simulink model "hexGroundContactTestHarness"  (R2024a)
settings: configuration reference "standardSILConfiguraitonParams" (kept outside this file)
undefined symbols (not defined in the file): vehicleParams
settings Model: Creator=jerem  LastModifiedBy=jerem
settings ConfigSetRef: SourceName=standardSILConfiguraitonParams  SourceLocation=Base Workspace

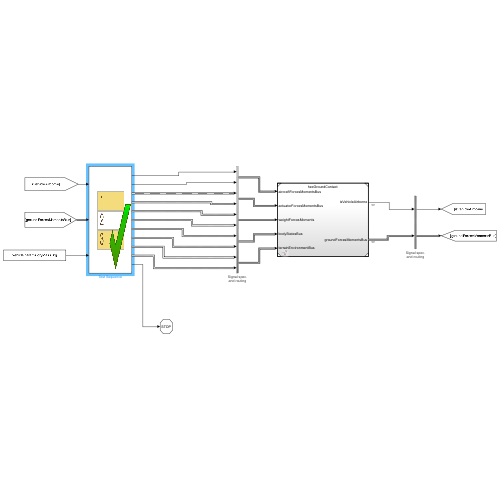
[thumbnail: Simulink's stored preview of the top-level diagram]
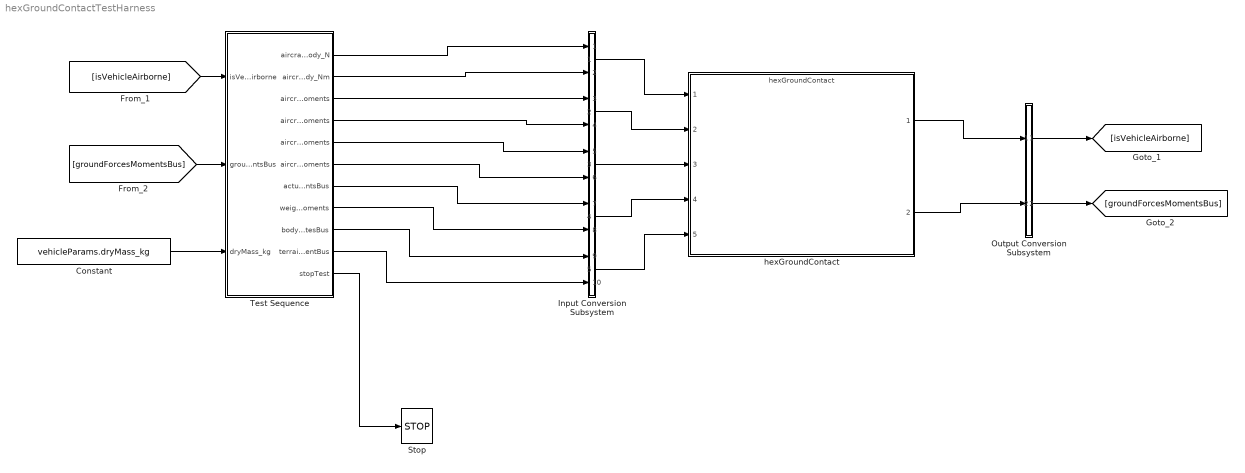
== system hexGroundContactTestHarness ==
  Constant : Constant  Value=vehicleParams.dryMass_kg
  Input Conversion Subsystem : Subsystem  Tag=__SLT_ICS__  Description=|
      | Signal spec.
      | and routing
      settings: AttributesFormatString=%<Description>
  Output Conversion Subsystem : Subsystem  Tag=__SLT_OCS__  Description=|
      | Signal spec.
      | and routing
      mask init:
      | ICDictionary = get_param(bdroot, 'DataDictionary');
      | if isempty(ICDictionary)
      |    ICScope = Simulink.data.BaseWorkspace;
      | else
      |    ICScope = Simulink.data.DataDictionary(ICDictionary);
      | end
      | 
      | IC2 = Simulink.Bus.createMATLABStruct('ComponentForcesMomentsBus', [], [1 1], ICScope);
      settings: AttributesFormatString=%<Description>
  Stop : Stop
  Test Sequence : Test Sequence  TreatAsAtomicUnit=on
  hexGroundContact : ModelReference  ModelNameDialog=hexGroundContact  SimulationMode=Normal  ModelReferenceVersion=1.58
  wires:
  Test Sequence/1(aircraftForcesMomentsBus_forcesInBody_N) -> Input Conversion Subsystem/1(Inport_1)
  Test Sequence/2(aircraftForcesMomentsBus_momentsInBody_Nm) -> Input Conversion Subsystem/2(Inport_2)
  Test Sequence/3(aircraftForcesMomentsBus_aeroForcesMoments) -> Input Conversion Subsystem/3(Inport_3)
  Test Sequence/4(aircraftForcesMomentsBus_engineForcesMoments) -> Input Conversion Subsystem/4(Inport_4)
  Test Sequence/5(aircraftForcesMomentsBus_groundForcesMoments) -> Input Conversion Subsystem/5(Inport_5)
  Test Sequence/6(aircraftForcesMomentsBus_weightForcesMoments) -> Input Conversion Subsystem/6(Inport_6)
  Test Sequence/7(actuatorForcesMomentsBus) -> Input Conversion Subsystem/7(Inport_7)
  Test Sequence/8(weightForcesMoments) -> Input Conversion Subsystem/8(Inport_8)
  Test Sequence/9(bodyStatesBus) -> Input Conversion Subsystem/9(Inport_9)
  Test Sequence/10(terrainEnvironmentBus) -> Input Conversion Subsystem/10(Inport_10)
  [isVehicleAirborne] -> Test Sequence/1(isVehicleAirborne)
  [groundForcesMomentsBus] -> Test Sequence/2(groundForcesMomentsBus)
  Output Conversion Subsystem/1(Outport_1) -> [isVehicleAirborne]
  Output Conversion Subsystem/2(Outport_2) -> [groundForcesMomentsBus]
  Input Conversion Subsystem/1(Outport_1) -> hexGroundContact/1
  Input Conversion Subsystem/2(Outport_2) -> hexGroundContact/2
  Input Conversion Subsystem/3(Outport_3) -> hexGroundContact/3
  Input Conversion Subsystem/4(Outport_4) -> hexGroundContact/4
  Input Conversion Subsystem/5(Outport_5) -> hexGroundContact/5
  hexGroundContact/1 -> Output Conversion Subsystem/1(Inport_1)
  hexGroundContact/2 -> Output Conversion Subsystem/2(Inport_2)
  Test Sequence/11(stopTest) -> Stop/1
  Constant/1 -> Test Sequence/3(dryMass_kg)

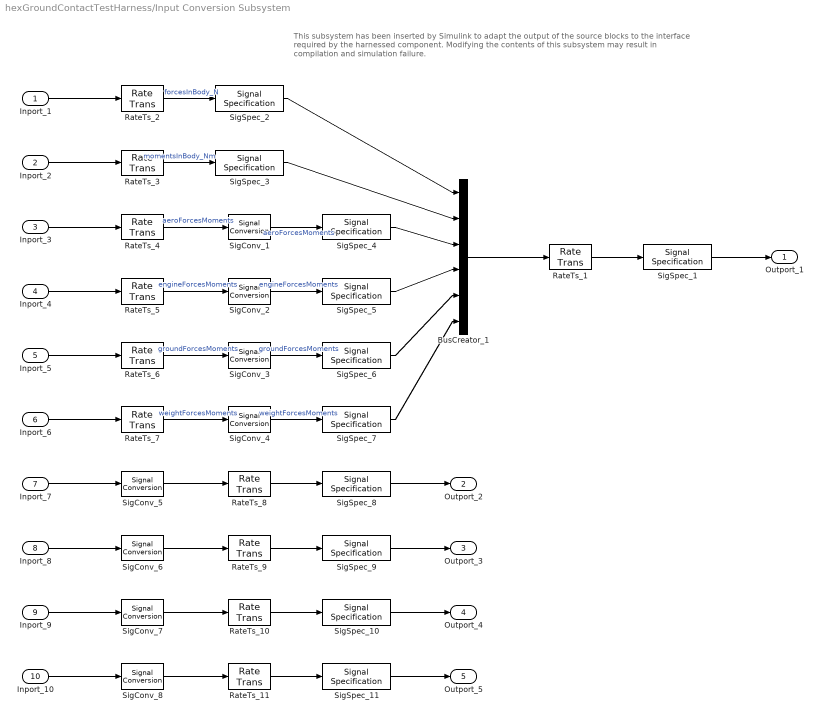
== system hexGroundContactTestHarness/Input Conversion Subsystem ==
  note: This subsystem has been inserted by Simulink to adapt the output of the source blocks to the interface required by the harnessed component.
      |  Modifying the contents of this subsystem may result in compilation and simulation failure.
  Inport_1 : Inport
  Inport_2 : Inport  Port=2
  Inport_3 : Inport  Port=3
  Inport_4 : Inport  Port=4
  Inport_5 : Inport  Port=5
  Inport_6 : Inport  Port=6
  Inport_7 : Inport  Port=7
  Inport_8 : Inport  Port=8
  Inport_9 : Inport  Port=9
  Inport_10 : Inport  Port=10
  BusCreator_1 : BusCreator  Inputs=6  OutDataTypeStr=Bus: AircraftForcesMomentsBus
  RateTs_{1..11} (11 alike) : RateTransition  OutPortSampleTime=0.004
  SigConv_{1..4} (4 alike) : SignalConversion  ConversionOutput=Nonvirtual bus  OverrideOpt=off
  SigConv_{5..8} (4 alike) : SignalConversion  ConversionOutput=Virtual bus  OverrideOpt=off
  SigSpec_1 : SignalSpecification  OutDataTypeStr=Bus: AircraftForcesMomentsBus  SampleTime=0.004
  SigSpec_10 : SignalSpecification  OutDataTypeStr=Bus: BodyStateBus  SampleTime=0.004
  SigSpec_11 : SignalSpecification  OutDataTypeStr=Bus: TerrainEnvironmentBus  SampleTime=0.004
  SigSpec_2 : SignalSpecification  OutDataTypeStr=double  Dimensions=[3]  SampleTime=0.004
  SigSpec_3 : SignalSpecification  OutDataTypeStr=double  Dimensions=[3]  SampleTime=0.004
  SigSpec_{4..7} (4 alike) : SignalSpecification  OutDataTypeStr=Bus: ComponentForcesMomentsBus  Dimensions=[1]  SampleTime=0.004  BusOutputAsStruct=on
  SigSpec_8 : SignalSpecification  OutDataTypeStr=Bus: ComponentForcesMomentsBus  SampleTime=0.004
  SigSpec_9 : SignalSpecification  OutDataTypeStr=Bus: ComponentForcesMomentsBus  SampleTime=0.004
  Outport_1 : Outport
  Outport_2 : Outport  Port=2
  Outport_3 : Outport  Port=3
  Outport_4 : Outport  Port=4
  Outport_5 : Outport  Port=5
  wires:
  SigSpec_1/1 -> Outport_1/1
  RateTs_1/1 -> SigSpec_1/1
  BusCreator_1/1 -> RateTs_1/1
  SigSpec_2/1 -> BusCreator_1/1
  RateTs_2/1 -> SigSpec_2/1  "forcesInBody_N"
  Inport_1/1 -> RateTs_2/1
  SigSpec_3/1 -> BusCreator_1/2
  RateTs_3/1 -> SigSpec_3/1  "momentsInBody_Nm"
  Inport_2/1 -> RateTs_3/1
  SigSpec_4/1 -> BusCreator_1/3
  SigConv_1/1 -> SigSpec_4/1  "aeroForcesMoments"
  RateTs_4/1 -> SigConv_1/1  "aeroForcesMoments"
  Inport_3/1 -> RateTs_4/1
  SigSpec_5/1 -> BusCreator_1/4
  SigConv_2/1 -> SigSpec_5/1  "engineForcesMoments"
  RateTs_5/1 -> SigConv_2/1  "engineForcesMoments"
  Inport_4/1 -> RateTs_5/1
  SigSpec_6/1 -> BusCreator_1/5
  SigConv_3/1 -> SigSpec_6/1  "groundForcesMoments"
  RateTs_6/1 -> SigConv_3/1  "groundForcesMoments"
  Inport_5/1 -> RateTs_6/1
  SigSpec_7/1 -> BusCreator_1/6
  SigConv_4/1 -> SigSpec_7/1  "weightForcesMoments"
  RateTs_7/1 -> SigConv_4/1  "weightForcesMoments"
  Inport_6/1 -> RateTs_7/1
  SigSpec_8/1 -> Outport_2/1
  RateTs_8/1 -> SigSpec_8/1
  SigConv_5/1 -> RateTs_8/1
  Inport_7/1 -> SigConv_5/1
  SigSpec_9/1 -> Outport_3/1
  RateTs_9/1 -> SigSpec_9/1
  SigConv_6/1 -> RateTs_9/1
  Inport_8/1 -> SigConv_6/1
  SigSpec_10/1 -> Outport_4/1
  RateTs_10/1 -> SigSpec_10/1
  SigConv_7/1 -> RateTs_10/1
  Inport_9/1 -> SigConv_7/1
  SigSpec_11/1 -> Outport_5/1
  RateTs_11/1 -> SigSpec_11/1
  SigConv_8/1 -> RateTs_11/1
  Inport_10/1 -> SigConv_8/1

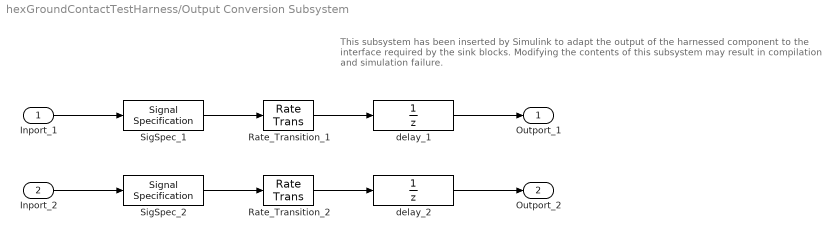
== system hexGroundContactTestHarness/Output Conversion Subsystem ==
  note: This subsystem has been inserted by Simulink to adapt the output of the harnessed component to the interface required by the sink blocks.
      |  Modifying the contents of this subsystem may result in compilation and simulation failure.
  Inport_1 : Inport
  Inport_2 : Inport  Port=2
  Rate_Transition_1 : RateTransition  OutPortSampleTimeOpt=Inherit
  Rate_Transition_2 : RateTransition  OutPortSampleTimeOpt=Inherit
  SigSpec_1 : SignalSpecification  OutDataTypeStr=boolean  Dimensions=[1]  SampleTime=0.004
  SigSpec_2 : SignalSpecification  OutDataTypeStr=Bus: ComponentForcesMomentsBus  Dimensions=[1]  SampleTime=0.004
  delay_1 : UnitDelay  SampleTime=-1
  delay_2 : UnitDelay  InitialCondition=IC2  SampleTime=-1
  Outport_1 : Outport
  Outport_2 : Outport  Port=2
  wires:
  Inport_1/1 -> SigSpec_1/1
  SigSpec_1/1 -> Rate_Transition_1/1
  Rate_Transition_1/1 -> delay_1/1
  delay_1/1 -> Outport_1/1
  Inport_2/1 -> SigSpec_2/1
  SigSpec_2/1 -> Rate_Transition_2/1
  Rate_Transition_2/1 -> delay_2/1
  delay_2/1 -> Outport_2/1

== stateflow chart hexGroundContactTestHarness/Test Sequence ==
  state Scenario_1
    state Initialize
      %% Initialize data outputs.
      aircraftForcesMomentsBus_forcesInBody_N = zeros(3, 1);
      aircraftForcesMomentsBus_momentsInBody_Nm = zeros(3, 1);
      aircraftForcesMomentsBus_aeroForcesMoments.forcesInBody_N = zeros(3,1);
      aircraftForcesMomentsBus_aeroForcesMoments.momentsInBody_Nm = zeros(3,1);
      aircraftForcesMomentsBus_engineForcesMoments.forcesInBody_N = zeros(3,1);
      aircraftForcesMomentsBus_engineForcesMoments.momentsInBody_Nm = zeros(3,1);
      aircraftForcesMomentsBus_groundForcesMoments.forcesInBody_N = zeros(3,1);
      aircraftForcesMomentsBus_groundForcesMoments.momentsInBody_Nm = zeros(3,1);
      aircraftForcesMomentsBus_weightForcesMoments.forcesInBody_N = zeros(3,1);
      aircraftForcesMomentsBus_weightForcesMoments.momentsInBody_Nm = zeros(3,1);
      actuatorForcesMomentsBus.forcesInBody_N = zeros(3,1);
      actuatorForcesMomentsBus.momentsInBody_Nm = zeros(3,1);
      weightForcesMoments.forcesInBody_N = zeros(3,1);
      weightForcesMoments.forcesInBody_N(3) = dryMass_kg * 9.81;
      weightForcesMoments.momentsInBody_Nm = zeros(3,1);
      bodyStatesBus.aircraftVelInNED_mps = zeros(3,1);
      bodyStatesBus.aircraftPosInNED_m = zeros(3,1);
      bodyStatesBus.aircraftEulerAngles_rad = zeros(3,1);
      bodyStatesBus.aircraftVelInBody_mps = zeros(3,1);
      bodyStatesBus.aircraftAngVelInBody_radps = zeros(3,1);
      bodyStatesBus.aircraftAngAccelInBody_radps2 = zeros(3,1);
      bodyStatesBus.aircraftAccelInBody_mps2 = zeros(3,1);
      bodyStatesBus.DCM_be = eye(3);
      bodyStatesBus.aircraftAccelbe_mps2 = zeros(3,1);
      terrainEnvironmentBus.terrainHeightInNED_m = 0;
      stopTest = false;
    state verifyNotMoving
      verify(isClose(bodyStatesBus.aircraftPosInNED_m(1),0))
      verify(isClose(bodyStatesBus.aircraftPosInNED_m(2),0))
      verify(isClose(bodyStatesBus.aircraftPosInNED_m(3),0))
      verify(isClose(groundForcesMomentsBus.forcesInBody_N(3), -dryMass_kg * 9.81))
      verify(~isVehicleAirborne)
      %Save the previous ground force, this will be used in the next verificaiton
      prevActuatorGroundForceZ_N = groundForcesMomentsBus.forcesInBody_N(3);
    state attemptToGoThroughFloor
      bodyStatesBus.aircraftAngVelInBody_radps(3) = 5; % Set aircraft velocity and force to go toward the ground
      actuatorForcesMomentsBus.forcesInBody_N(3) = 10;
    state verifyVehicleNotGoingThroughGround
      verify(prevActuatorGroundForceZ_N >  groundForcesMomentsBus.forcesInBody_N(3)) % Ground should be applying larger -Z force (pointing up toward the sky)
    state setVehicleAirborne
      bodyStatesBus.aircraftPosInNED_m(3) = -10;
    state verifyVehicleIsAirborne
      verify(isVehicleAirborne)
      verify(isClose(groundForcesMomentsBus.forcesInBody_N(1),0))
      verify(isClose(groundForcesMomentsBus.forcesInBody_N(2),0))
      verify(isClose(groundForcesMomentsBus.forcesInBody_N(3),0))
    state EndTest
      stopTest = true;
    (default) -> Initialize
    Initialize -> verifyNotMoving : [
        | true
        | ]
    verifyNotMoving -> attemptToGoThroughFloor : [
        | after(1,sec)
        | ]
    attemptToGoThroughFloor -> verifyVehicleNotGoingThroughGround : [
        | after(1,sec)
        | ]
    verifyVehicleNotGoingThroughGround -> setVehicleAirborne : [
        | after(1,tick)
        | ]
    setVehicleAirborne -> verifyVehicleIsAirborne : [
        | after(1,sec)
        | ]
    verifyVehicleIsAirborne -> EndTest : [
        | after(1,tick)
        | ]
  (default) -> Scenario_1 : {assert(Active_Scenario_Index == 1,'The value of Scenario Parameter ''Active_Scenario_Index'' is not valid. Use the index of the scenario to specify it.')}
  data: isVehicleAirborne input boolean size=[1]; groundForcesMomentsBus input Bus: ComponentForcesMomentsBus size=[1]; aircraftForcesMomentsBus_forcesInBody_N output double size=[3]; aircraftForcesMomentsBus_momentsInBody_Nm output double size=[3]; aircraftForcesMomentsBus_aeroForcesMoments output Bus: ComponentForcesMomentsBus size=[1]; aircraftForcesMomentsBus_engineForcesMoments output Bus: ComponentForcesMomentsBus size=[1]; aircraftForcesMomentsBus_groundForcesMoments output Bus: ComponentForcesMomentsBus size=[1]; aircraftForcesMomentsBus_weightForcesMoments output Bus: ComponentForcesMomentsBus size=[1]; actuatorForcesMomentsBus output Bus: ComponentForcesMomentsBus size=[1]; weightForcesMoments output Bus: ComponentForcesMomentsBus size=[1]; bodyStatesBus output Bus: BodyStateBus size=[1]; terrainEnvironmentBus output Bus: TerrainEnvironmentBus size=[1]; stopTest output; Active_Scenario_Index parameter =1; dryMass_kg input; prevActuatorGroundForceZ_N local
